simulink model "DynamicsModel2"  (R2019a)
settings: Solver=ode45  StartTime=0.0  StopTime=400  MaxStep=2.0  RelTol=1e-3
libraries: simulink x2, aerolibatmos2 x1
settings Model: Creator=Daniel  LastModifiedBy=Daniel

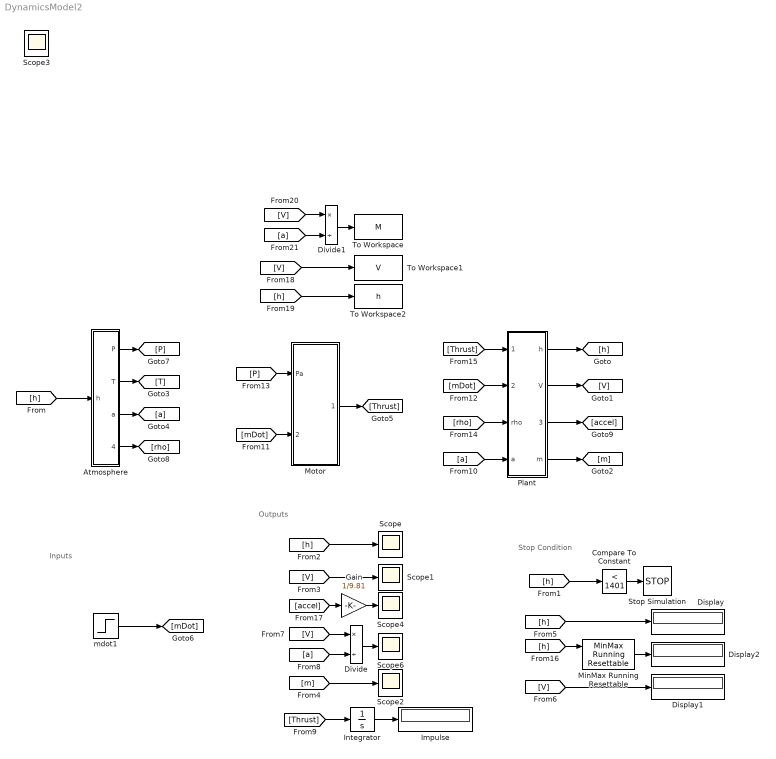
== system DynamicsModel2 ==
  note: Stop Condition
  note: Outputs
  note: Inputs
  Atmosphere : Subsystem
  Compare To Constant : simulink/Logic and Bit Operations/Compare To Constant  relop=<  const=1401  OutDataTypeStr=boolean
  Display : Display
  Display1 : Display
  Display2 : Display
  Divide : Product  Inputs=*/
  Divide1 : Product  Inputs=*/
  Gain : Gain  Gain=1/9.81
  Impulse : Display
  Integrator : Integrator
  MinMax Running Resettable : simulink/Math Operations/MinMax Running Resettable  Function=max  vinit=0.0
  Motor : Subsystem
  Plant : Subsystem
  Scope{,1..4,6} (6 alike) : Scope
  Stop Simulation : Stop
  To Workspace : ToWorkspace  VariableName=M  SaveFormat=Timeseries  SampleTime=-1
  To Workspace1 : ToWorkspace  VariableName=V  SaveFormat=Timeseries  SampleTime=-1
  To Workspace2 : ToWorkspace  VariableName=h  SaveFormat=Timeseries  SampleTime=-1
  mdot1 : Step  Time=72  Before=5  After=0  SampleTime=0
  wires:
  [mDot] -> Motor/2(mDot)
  Motor/1(Thrust) -> [Thrust]
  Compare To Constant/1 -> Stop Simulation/1
  Plant/1(h) -> [h]
  Plant/2(V) -> [V]
  [h] -> Compare To Constant/1
  Plant/4(m) -> [m]
  [h] -> Scope/1
  [V] -> Scope1/1
  [m] -> Scope2/1
  Integrator/1 -> Impulse/1
  [h] -> Atmosphere/1(h)
  Atmosphere/3(a) -> [a]
  Atmosphere/2(T) -> [T]
  [V] -> Divide/1
  [a] -> Divide/2
  Divide/1 -> Scope6/1
  [Thrust] -> Integrator/1
  [a] -> Plant/4(a)
  mdot1/1 -> [mDot]
  [mDot] -> Plant/2(mdot)
  Atmosphere/1(P) -> [P]
  [P] -> Motor/1(Pa)
  Atmosphere/4(rho) -> [rho]
  [rho] -> Plant/3(rho)
  [Thrust] -> Plant/1("Thrust ")
  [h] -> Display/1
  [V] -> Display1/1
  [h] -> MinMax Running Resettable/1
  MinMax Running Resettable/1 -> Display2/1
  Plant/3(accel) -> [accel]
  [accel] -> Gain/1
  Gain/1 -> Scope4/1
  Divide1/1 -> To Workspace/1
  [a] -> Divide1/2
  [V] -> Divide1/1
  [V] -> To Workspace1/1
  [h] -> To Workspace2/1

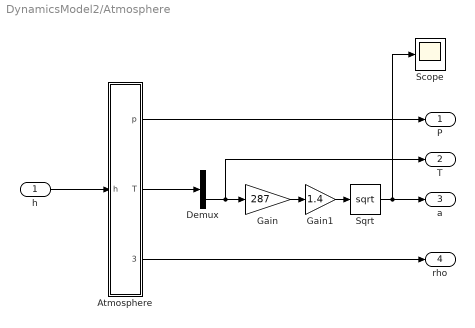
== system DynamicsModel2/Atmosphere ==
  h : Inport
  Atmosphere : Subsystem
  Demux : Demux  Outputs=2
  Gain : Gain  Gain=287
  Gain1 : Gain  Gain=1.4
  Scope : Scope
  Sqrt : Sqrt  SaturateOnIntegerOverflow=on
  P : Outport
  T : Outport  Port=2
  a : Outport  Port=3
  rho : Outport  Port=4
  wires:
  Sqrt/1 -> Scope/1, a/1
  h/1 -> Atmosphere/1(h)
  Atmosphere/1(p) -> P/1
  Demux/2 -> T/1, Gain/1
  Gain/1 -> Gain1/1
  Atmosphere/2(T) -> Demux/1
  Atmosphere/3(rho) -> rho/1
  Gain1/1 -> Sqrt/1

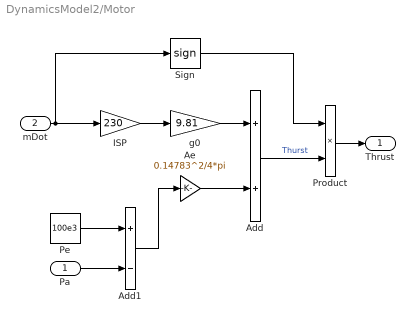
== system DynamicsModel2/Motor ==
  Pa : Inport
  mDot : Inport  Port=2
  Add : Sum
  Add1 : Sum  Inputs=+-
  Ae : Gain  Gain=0.14783^2/4*pi
  ISP : Gain  Gain=230
  Pe : Constant  Value=100e3
  Product : Product
  Sign : Signum
  g0 : Gain  Gain=9.81
  Thrust : Outport
  wires:
  Pe/1 -> Add1/1
  mDot/1 -> ISP/1, Sign/1
  Pa/1 -> Add1/2
  Ae/1 -> Add/2
  Sign/1 -> Product/1
  Add/1 -> Product/2  "Thurst"
  Add1/1 -> Ae/1
  Product/1 -> Thrust/1
  g0/1 -> Add/1
  ISP/1 -> g0/1

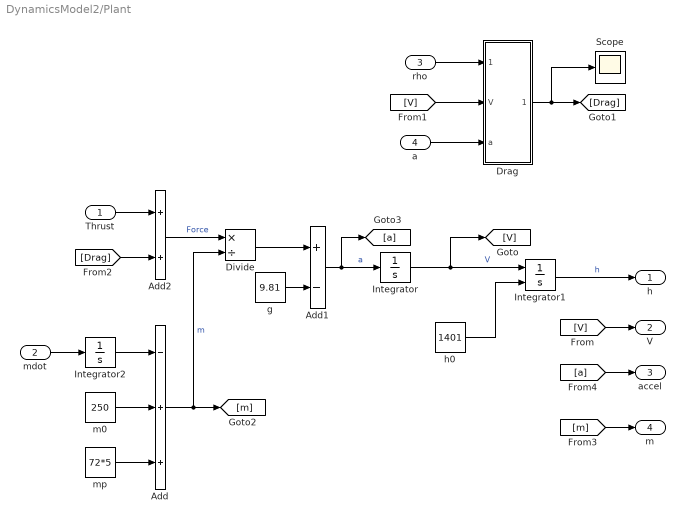
== system DynamicsModel2/Plant ==
  "Thrust " : Inport
  mdot : Inport  Port=2
  rho : Inport  Port=3
  a : Inport  Port=4
  Add : Sum  Inputs=-++
  Add1 : Sum  Inputs=+-
  Add2 : Sum
  Divide : Product  Inputs=*/
  Drag : Subsystem
  Integrator : Integrator
  Integrator1 : Integrator  InitialConditionSource=external
  Integrator2 : Integrator
  Scope : Scope
  g : Constant  Value=9.81
  h0 : Constant  Value=1401
  m0 : Constant  Value=250
  mp : Constant  Value=72*5
  h : Outport
  V : Outport  Port=2
  accel : Outport  Port=3
  m : Outport  Port=4
  wires:
  Integrator1/1 -> h/1  "h"
  Integrator/1 -> [V], Integrator1/1  "V"
  Add/1 -> [m], Divide/2  "m"
  Divide/1 -> Add1/1
  Add1/1 -> [a], Integrator/1  "a"
  [V] -> V/1
  g/1 -> Add1/2
  Add2/1 -> Divide/1  "Force"
  "Thrust "/1 -> Add2/1
  [Drag] -> Add2/2
  Integrator2/1 -> Add/1
  rho/1 -> Drag/1(Rho)
  [m] -> m/1
  mdot/1 -> Integrator2/1
  [V] -> Drag/2(V)
  mp/1 -> Add/3
  m0/1 -> Add/2
  a/1 -> Drag/3(a)
  h0/1 -> Integrator1/2
  Drag/1(Drag) -> Scope/1, [Drag]
  [a] -> accel/1

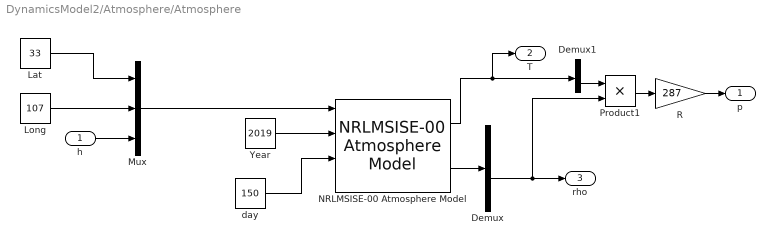
== system DynamicsModel2/Atmosphere/Atmosphere ==
  h : Inport
  Demux : Demux  Outputs=9
  Demux1 : Demux  Outputs=2
  "Lat " : Constant  Value=33
  Long : Constant  Value=107
  Mux : Mux  Inputs=3
  NRLMSISE-00 Atmosphere Model : aerolibatmos2/NRLMSISE-00 Atmosphere Model  units=Metric (MKS)  lst_input=off  flux_ap_input=off  flags_input=Internal  flags=ones(1,23)  oxygen_in=off  action=Warning
      settings: SourceProductName=Aerospace Blockset  SourceProductBaseCode=AE
  Product1 : Product
  R : Gain  Gain=287
  Year : Constant  Value=2019
  day : Constant  Value=150
  p : Outport
  T : Outport  Port=2
  rho : Outport  Port=3
  wires:
  Demux/6 -> rho/1, Product1/2
  Demux1/2 -> Product1/1
  "Lat "/1 -> Mux/1
  Product1/1 -> R/1
  day/1 -> NRLMSISE-00 Atmosphere Model/3
  Long/1 -> Mux/2
  Mux/1 -> NRLMSISE-00 Atmosphere Model/1
  NRLMSISE-00 Atmosphere Model/2 -> Demux/1
  R/1 -> p/1
  Year/1 -> NRLMSISE-00 Atmosphere Model/2
  NRLMSISE-00 Atmosphere Model/1 -> T/1, Demux1/1
  h/1 -> Mux/3

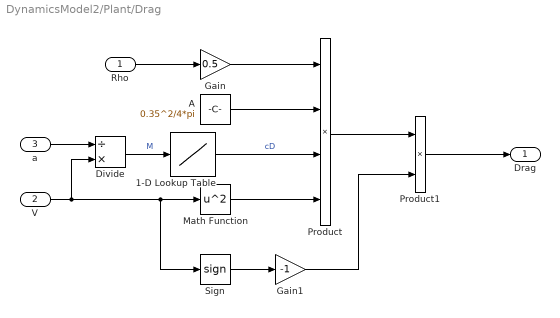
== system DynamicsModel2/Plant/Drag ==
  Rho : Inport
  V : Inport  Port=2
  a : Inport  Port=3
  1-D Lookup Table : Lookup_n-D  NumberOfTableDimensions=1  BreakpointsSpecification=Even spacing  BreakpointsForDimension1=[-5:5]  BreakpointsForDimension1FirstPoint=0.1  BreakpointsForDimension1Spacing=0.1  Table=CDvsMach(2:end, 2)  InternalRulePriority=Speed  RndMeth=Simplest  InputSameDT=on
  A : Constant  Value=0.35^2/4*pi
  Divide : Product  Inputs=/*
  Gain : Gain  Gain=0.5
  Gain1 : Gain  Gain=-1
  Math Function : Math  Operator=square  SaturateOnIntegerOverflow=on
  Product : Product  Inputs=4
  Product1 : Product
  Sign : Signum
  Drag : Outport
  wires:
  Gain/1 -> Product/1
  Math Function/1 -> Product/4
  V/1 -> Sign/1, Math Function/1, Divide/2
  Rho/1 -> Gain/1
  A/1 -> Product/2
  Product/1 -> Product1/1
  Product1/1 -> Drag/1
  Sign/1 -> Gain1/1
  Gain1/1 -> Product1/2
  a/1 -> Divide/1
  Divide/1 -> 1-D Lookup Table/1  "M"
  1-D Lookup Table/1 -> Product/3  "cD"
